simulink model "countertest"  (R2017b)
settings: Solver=VariableStepAuto  StartTime=0.0  StopTime=inf  RelTol=1e-3
settings Model: Creator=E6320  LastModifiedBy=E6320

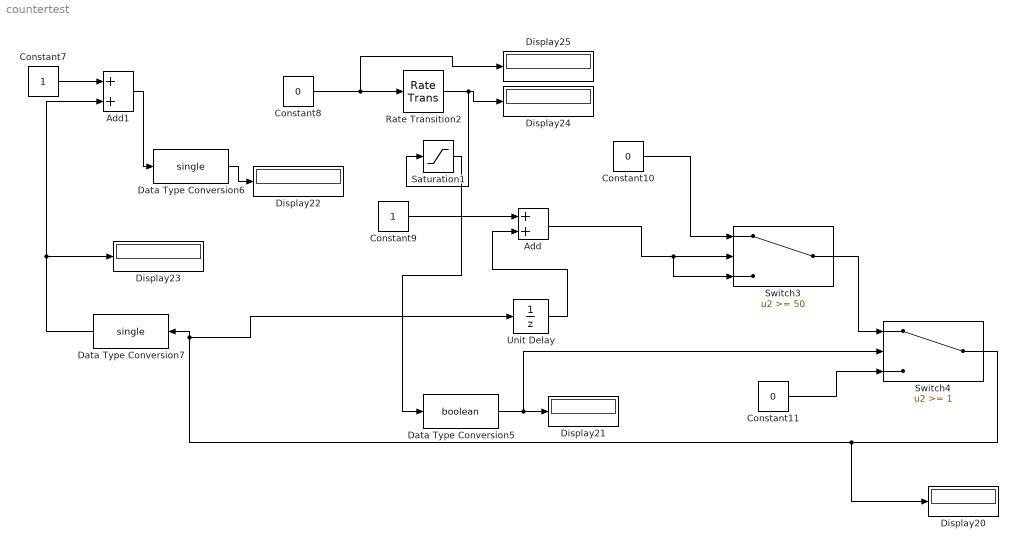
== system countertest ==
  Add : Sum  OutDataTypeStr=single
  Add1 : Sum  OutDataTypeStr=single  RndMeth=Ceiling
  Constant10 : Constant  Value=0
  Constant11 : Constant  Value=0
  Constant7 : Constant  OutDataTypeStr=single
  Constant8 : Constant  Value=0  OutDataTypeStr=single
  Constant9 : Constant  OutDataTypeStr=boolean
  Data Type Conversion5 : DataTypeConversion  OutDataTypeStr=boolean
  Data Type Conversion6 : DataTypeConversion  OutDataTypeStr=single  RndMeth=Round
  Data Type Conversion7 : DataTypeConversion  OutDataTypeStr=single  RndMeth=Ceiling
  Display{20..25} (6 alike) : Display
  Rate Transition2 : RateTransition  OutPortSampleTime=1
  Saturation1 : Saturate  UpperLimit=1  LowerLimit=0
  Switch3 : Switch  Threshold=50
  Switch4 : Switch  Threshold=1
  Unit Delay : UnitDelay  InputProcessing=Columns as channels (frame based)
  wires:
  Add/1 -> Switch3/3, Switch3/2
  Constant11/1 -> Switch4/3
  Constant10/1 -> Switch3/1
  Data Type Conversion7/1 -> Display23/1, Add1/2
  Data Type Conversion6/1 -> Display22/1
  Switch3/1 -> Switch4/1
  Add1/1 -> Data Type Conversion6/1
  Unit Delay/1 -> Add/2
  Rate Transition2/1 -> Saturation1/1, Display24/1
  Switch4/1 -> Display20/1, Unit Delay/1, Data Type Conversion7/1
  Data Type Conversion5/1 -> Switch4/2, Display21/1
  Constant7/1 -> Add1/1
  Constant9/1 -> Add/1
  Constant8/1 -> Display25/1, Rate Transition2/1
  Saturation1/1 -> Data Type Conversion5/1
